simulink model "pp_rob2_c_ss"  (Simulink 5.0)
settings: Solver=ode23s  StartTime=t0  StopTime=tf  RelTol=1e-8  AbsTol=1.0e-8
values from neighbouring files (symbols this model uses):
  a = [0 1 0; a21 0 a23; 0 0 a33]    [ball_im.m]    (also in ball_opt.m; ball_psi.m)
  b = [0; 0; b3]    [ball_im.m]    (also in ball_opt.m; ball_psi.m)
  c = [1 0 0]    [ball_im.m]    (also in ball_opt.m; ball_psi.m)
  d = 0    [ball_im.m]    (also in ball_opt.m; ball_psi.m)
  Delta = [1 -1]    [ball_im.m]    (also in endsem_06.m; pid_neg.m; pp_im_high.m = 1)
  R = 1    [ball_im.m]    (also in ball_opt.m; ball_psi.m; pp_im_high.m = conv(Bg,R1); pp_opt.m = conv(Bg,R1))
  S = conv(Ag,S1)    [pp_im_high.m]    (also in pp_opt.m; pp_psi-sav.m)
  st = 0.0001    [ball_im.m]    (also in ball_opt.m; ball_psi.m; comb.m = 1; endsem_06.m = 1)
  TM = gamma*T    [comb.m]
  Ts = 0.01; [B,A,k] = myc2d(G,Ts)    [ball_im.m]    (also in ball_opt.m; ball_psi.m; comb.m = 0.001; endsem_06.m = 1)
  xInitial = [0 0 0]    [ball_im.m]    (also in ball_opt.m; ball_psi.m; endsem_06.m = [0 0])
settings Model: Creator=kannanm  LastModifiedBy=kannan  ExtModeAutoUpdateStatusClock=off

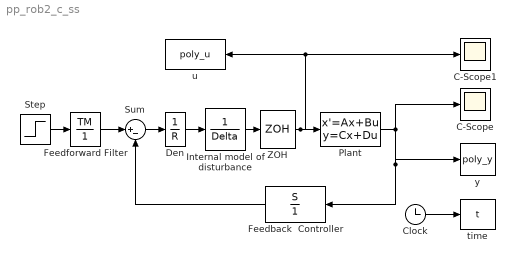
== system pp_rob2_c_ss ==
  C-Scope : Scope
      settings: YMin=0  YMax=1.2
  C-Scope1 : Scope
      settings: YMin=0  YMax=1.2
  Clock : Clock
      settings: Decimation=10
  Den : DiscreteFilter  Numerator=1  Denominator=R  SampleTime=Ts
  Feedback  Controller : DiscreteFilter  Orientation=left  Numerator=S  Denominator=1  SampleTime=Ts
  Feedforward Filter : DiscreteFilter  Numerator=TM  Denominator=1  SampleTime=Ts
  Internal model of disturbance : DiscreteFilter  Numerator=1  Denominator=Delta  SampleTime=Ts
  Plant : StateSpace  A=a  B=b  C=c  D=d  X0=xInitial
  Step : Step  Time=0  After=st  SampleTime=Ts
  Sum : Sum  Inputs=|+-  SaturateOnIntegerOverflow=on
  ZOH : ZeroOrderHold  SampleTime=Ts
  time : ToWorkspace  VariableName=t  SampleTime=Ts  SaveFormat=Array
  u : ToWorkspace  VariableName=poly_u  SampleTime=Ts  SaveFormat=Array
  y : ToWorkspace  VariableName=poly_y  SampleTime=Ts  SaveFormat=Array
  wires:
  Step/1 -> Feedforward Filter/1
  Feedforward Filter/1 -> Sum/1
  Sum/1 -> Den/1
  Feedback  Controller/1 -> Sum/2
  ZOH/1 -> Plant/1, u/1, C-Scope1/1
  Clock/1 -> time/1
  Plant/1 -> Feedback  Controller/1, y/1, C-Scope/1
  Internal model of disturbance/1 -> ZOH/1
  Den/1 -> Internal model of disturbance/1
